simulink model "ChirpBeatfreq"  (R2025b)
settings: Solver=FixedStepAuto  StartTime=0.0  StopTime=5  RelTol=1e-3
libraries: dspfdesign x1, dspsrcs4 x1
settings Model: Creator=Amrut  LastModifiedBy=Amrut

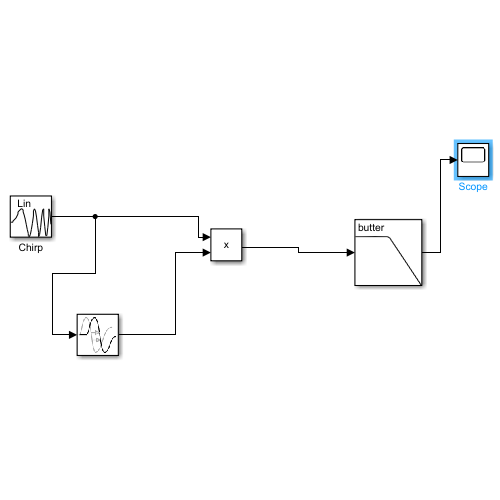
[thumbnail: Simulink's stored preview of the top-level diagram]
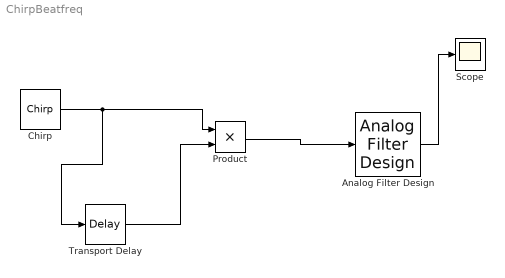
== system ChirpBeatfreq ==
  Analog Filter Design : dspfdesign/Analog Filter Design  method=Butterworth  filttype=Lowpass  N=8  Wlo=500e3  Whi=80  Rp=2  Rs=40
  Chirp : dspsrcs4/Chirp  sweep=Linear  mode=Unidirectional  f0=1000  f1=4000  t1=1  Tsweep=1  phase=0  Ts=1/2e6  spf=1  datatype=double  OutputFrames=off
  Product : Product
  Scope : Scope
      settings: ActiveDisplayYMinimum=-0.10083327685543486  ActiveDisplayYMaximum=1.2878832561426159
  Transport Delay : TransportDelay  DelayTime=1e-6
  wires:
  Chirp/1 -> Transport Delay/1, Product/1
  Transport Delay/1 -> Product/2
  Product/1 -> Analog Filter Design/1
  Analog Filter Design/1 -> Scope/1
